simulink model "cellModel"  (Simulink 9.1)
settings: Solver=ode1  StartTime=0.0  StopTime=Tend  FixedStep=1  RelTol=1e-3  EnableMultiTasking=on
values from neighbouring files (symbols this model uses):
  beta = 1/(R*C)    (= 0.184556326591)    [ElectricCircuit_Model_Batt.m]    (also in ElectricCircuit_Model_Batt_Original.m; Error_R0.m = 1/(R*C); Error_R0_original.m)
  capacity = 2.15596073014    [Midterm_Data_Testing.mat]    (also in batt_parameters.mat = 2.2163325381)
  e0 = [2.84172372701 3.1116289636 3.22991808698 3.31134692108 3.37184040482 3.40917768947 3.423922705 3.43211244396 3.43833083131 3.44368103281 3.44851066715 3.453021097 ... (101 elements, 101x1)]    [Midterm_Data_Testing.mat]    (also in batt_parameters.mat = [2.7145326117 2.78349893959 2.84397506836 2.89701380592 2.94)
  gamma = 1/C    (= 0.000959692898273)    [ElectricCircuit_Model_Batt.m]    (also in ElectricCircuit_Model_Batt_Original.m; Error_R0.m = 1/C; Error_R0_original.m)
  initialSoC = 1    [Midterm_Data_Testing.mat]    (also in batt_parameters.mat = 0.5)
  r0 = R0opt; sim('cellModel_R2016a',[Tend])    [ElectricCircuit_Model_Batt.m]    (also in ElectricCircuit_Model_Batt_Original.m; Error_R0.m = x(1); Error_R0_original.m = x)
libraries: simulink x1
settings Model: SuppressorTable=22 serialization::archive 11 0 6 0 0 0 0 0  Creator=Onori
settings DataIOCC: LimitDataPoints=on  SignalLoggingSaveFormat=ModelDataLogs
settings OptimizationCC: ExpressionDepthLimit=2147483647
settings DebuggingCC: SolverPrmCheckMsg=warning  FcnCallInpInsideContextMsg=warning  StateNameClashWarn=warning
settings GRTTargetCC: GeneratePreprocessorConditionals=Disable all  CombineOutputUpdateFcns=on  GRTInterface=off

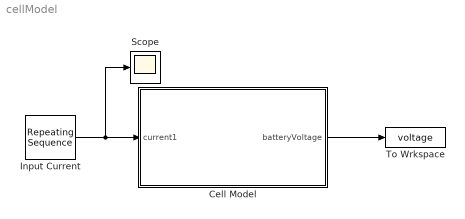
== system cellModel ==
  Cell Model : Subsystem
  Input Current : simulink/Sources/Repeating Sequence  rep_seq_t=t_data  rep_seq_y=I_data
  Scope : Scope
  To Wrkspace : ToWorkspace  VariableName=voltage  SampleTime=-1
  wires:
  Cell Model/1(batteryVoltage) -> To Wrkspace/1
  Input Current/1 -> Scope/1, Cell Model/1(current1)

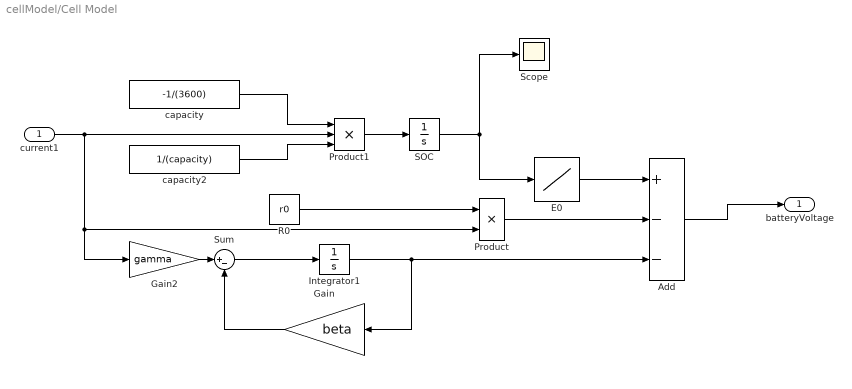
== system cellModel/Cell Model ==
  current1 : Inport
  Add : Sum  Inputs=+--
  E0 : Lookup_n-D  NumberOfTableDimensions=1  BreakpointsForDimension1=linspace(0,1,length(e0))  Table=e0  RndMeth=Simplest  InputSameDT=on
  Gain : Gain  Gain=beta
  Gain2 : Gain  Gain=gamma
  Integrator1 : Integrator
  Product : Product  RndMeth=Zero
  Product1 : Product  Inputs=3  RndMeth=Zero
  R0 : Constant  Value=r0
  SOC : Integrator  InitialCondition=initialSoC
  Scope : Scope
  Sum : Sum  Inputs=|+-
  capacity : Constant  Value=-1/(3600)
  capacity2 : Constant  Value=1/(capacity)
  batteryVoltage : Outport
  wires:
  current1/1 -> Product1/2, Gain2/1, Product/2
  capacity2/1 -> Product1/3
  E0/1 -> Add/1
  R0/1 -> Product/1
  Product/1 -> Add/2
  Add/1 -> batteryVoltage/1
  capacity/1 -> Product1/1
  Product1/1 -> SOC/1
  Gain2/1 -> Sum/1
  Sum/1 -> Integrator1/1
  SOC/1 -> Scope/1, E0/1
  Integrator1/1 -> Gain/1, Add/3
  Gain/1 -> Sum/2
